simulink model "esercizio_3_massaMollaSmorzatore"  (R2024a)
settings: Solver=FixedStepAuto  StartTime=0.0  StopTime=15  RelTol=1e-3
PreLoadFcn:
  | clear %%pulisce il workspace
  | 
  | % --------------------
  | % system's parameters:
  | % --------------------
  | 
  | M = 5 % massa
  | M_nominal = M
  | K = 5 % costante elastica
  | K_nominal = K
  | S = 5 % costante smorzatore
  | S_nominal = S
  | 
  | N = 5 % numero giunti intere molla
  | L = 10 % lunghezza giunti
  | 
  | % --------------------
  | % desired eigenvalues
  | % --------------------
  | eig_H = 2*[-1 -2 ]
  | eig_G = 1*[-1 -2 ]
  | 
  | % --------------------
  | % matrix and initial conditions
  | % --------------------
  | A = [   0     1    ;
  |       -K/M  -S/M   ]
  | 
  | 
  | B = [  0  ;
  |       1/M ]
  | 
  | 
  | C = [0 1]
  | 
  | D = zeros(size(C,1),size(B,2))
  | 
  | 
  | dimx = size(A,1)  % quindi dimx = 2
  | dimu = size(B,2)  % quindi dimu = 1
  | dimy = size(C,1)  % quindi dimy = 1
  | 
  | x0 = [15; % posizione iniziale
  |       20] % velocità iniziale
  | % x0 = [0 0 0 0]'; %p.to di equilibrio
  | 
  | % --------------------
  | % certainty-equivalence state-feedback controller
  | % --------------------
  | G=place(A,B,eig_G) % costruisce matrice G dati gli autovalori desiderati
  | 
  | % --------------------
  | % Luenberger observer
  | % --------------------
  | 
  | %luenberger obs:
  | %  z_dot = Az + Bu + H(y-Cz) = (A-HC)z +[B H] [u y]
  | 
  | % initial conditions
  | z0 = [-.5; % posizione iniziale stimata
  |       -.31] % velocità iniziale stimata
  | 
  | %z0 = x0  %partenza con stima ok
  | 
  | H=place(A',C',eig_H)' % costruisce matrice H dati gli autovalori desiderati
  | 
  | A_lu = A-H*C
  | 
  | B_lu = [B H]
  | 
  | C_lu = eye(size(A))
  | 
  | D_lu = zeros(size(C_lu,1),size(B_lu,2))
InitFcn:
  | % --------------------
  | % matrix and initial conditions
  | % --------------------
  | A = [   0     1    ;
  |       -K_nominal/M_nominal  -S_nominal/M_nominal   ]
  | 
  | 
  | B = [  0  ;
  |       1/M_nominal ]
  | 
  | 
  | C = [ 0 1 ]
  | 
  | D = zeros(size(C,1),size(B,2))
  | 
  | % --------------------
  | % certainty-equivalence state-feedback controller
  | % --------------------
  | G=place(A,B,eig_G) % costruisce matrice G dati gli autovalori desiderati
  | 
  | % --------------------
  | % Luenberger observer
  | % --------------------
  | 
  | H=place(A',C',eig_H)' % costruisce matrice H dati gli autovalori desiderati
  | 
  | A_lu = A-H*C
  | 
  | B_lu = [B H]
  | 
  | C_lu = eye(size(A))
  | 
  | D_lu = zeros(size(C_lu,1),size(B_lu,2))
libraries: vrlib x14, sldrtlib x1
settings Model: Creator=39342  LastModifiedBy=39342

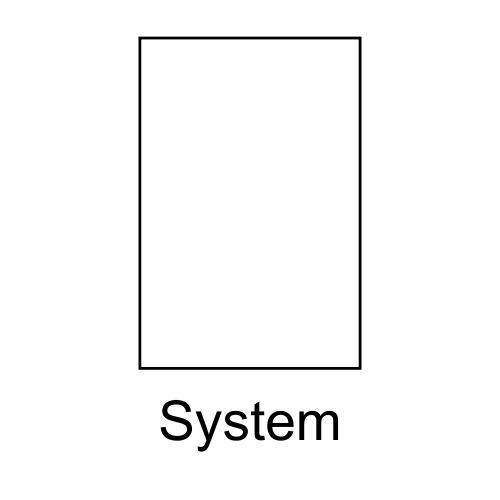
[thumbnail: Simulink's stored preview of the top-level diagram]
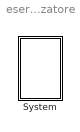
== system esercizio_3_massaMollaSmorzatore ==
  System : Subsystem

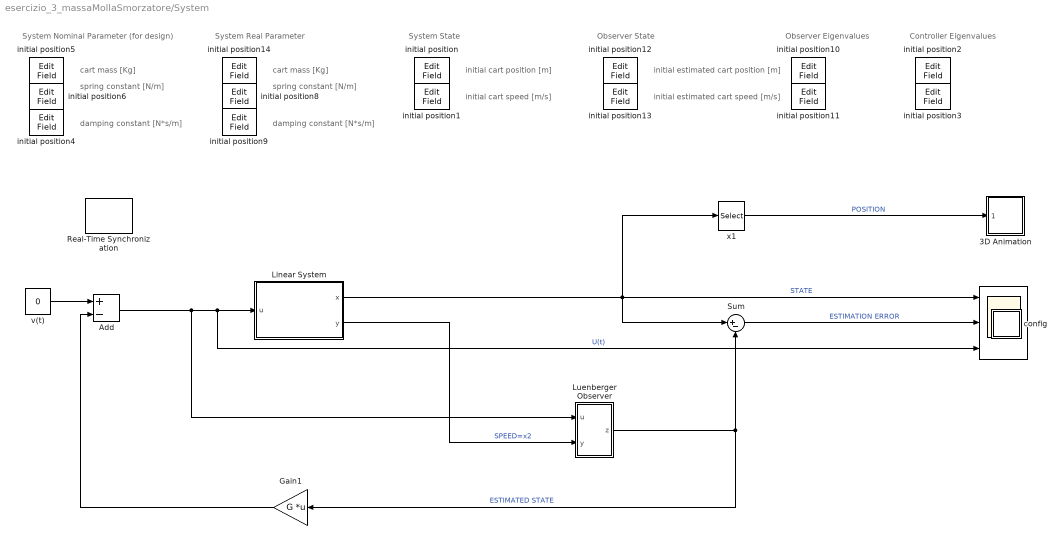
== system esercizio_3_massaMollaSmorzatore/System ==
  note: spring constant [N/m]
  note: initial estimated cart speed [m/s]
  note: System Real Parameter
  note: initial cart speed [m/s]
  note: cart mass [Kg]
  note: damping constant [N*s/m]
  note: initial cart position [m]
  note: Controller Eigenvalues
  note: cart mass [Kg]
  note: System State
  note: initial estimated cart position [m]
  note: damping constant [N*s/m]
  note: System Nominal Parameter (for design)
  note: Observer State
  note: Observer Eigenvalues
  note: spring constant [N/m]
  "     " : Scope  NumInputPorts=3
  3D Animation : Subsystem
  Add : Sum  Inputs=+-
  Gain1 : Gain  Gain=G  Multiplication=Matrix(K*u)
  Linear System : Subsystem
  Luenberger Observer : Subsystem
  Real-Time Synchronization : sldrtlib/Real-Time Synchronization  SampleTime=0.01  MaxMissedTicks=500  ShowMissedTicks=off  YieldWhenWaiting=off
  Sum : Sum  Inputs=|+-
  config : Subsystem
  initial position{,1..6,8..14} (14 alike) : EditField  LabelPosition=Hide  ShowInitialText=on  Alignment=Center
  v(t) : Constant  Value=0
  x1 : Selector  InputPortWidth=2  IndexOptions=Index vector (dialog)  Indices=[1]  OutputSizes=1
  wires:
  Sum/1 -> "     "/2  "ESTIMATION ERROR"
  x1/1 -> 3D Animation/1(position)  "POSITION"
  v(t)/1 -> Add/1
  Gain1/1 -> Add/2
  Luenberger Observer/1(z) -> Gain1/1, Sum/2  "ESTIMATED STATE"
  Linear System/1(x) -> Sum/1, "     "/1, x1/1  "STATE"
  Linear System/2(y) -> Luenberger Observer/2(y)  "SPEED=x2"
  Add/1 -> Linear System/1(u), "     "/3, Luenberger Observer/1(u)  "U(t)"

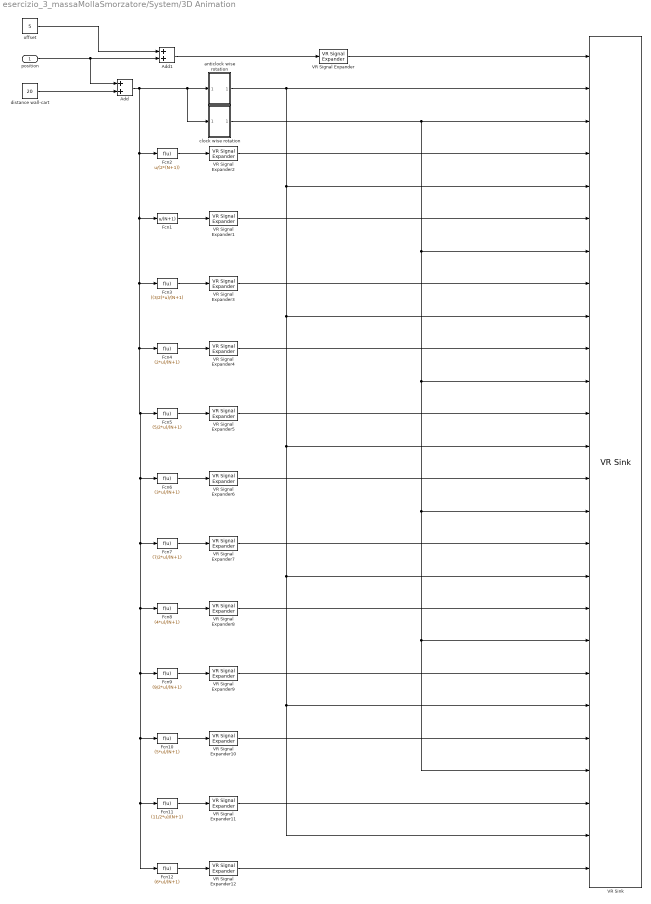
== system esercizio_3_massaMollaSmorzatore/System/3D Animation ==
  position : Inport
  Add : Sum
  Add1 : Sum
  Fcn1 : Fcn  Expr=u/(N+1)
  Fcn10 : Fcn  Expr=(5*u)/(N+1)
  Fcn11 : Fcn  Expr=(11/2*u)/(N+1)
  Fcn12 : Fcn  Expr=(6*u)/(N+1)
  Fcn2 : Fcn  Expr=u/(2*(N+1))
  Fcn3 : Fcn  Expr=((3/2)*u)/(N+1)
  Fcn4 : Fcn  Expr=(2*u)/(N+1)
  Fcn5 : Fcn  Expr=(5/2*u)/(N+1)
  Fcn6 : Fcn  Expr=(3*u)/(N+1)
  Fcn7 : Fcn  Expr=(7/2*u)/(N+1)
  Fcn8 : Fcn  Expr=(4*u)/(N+1)
  Fcn9 : Fcn  Expr=(9/2*u)/(N+1)
  VR Signal Expander{,1..12} (13 alike) : vrlib/VR Signal Expander  outwidth=3  outidx=[1]
  VR Sink : vrlib/VR Sink  InstantiateOnLoad=on  SampleTime=0.1  ViewEnable=on  RemoteChange=off  RemoteView=off  FieldsWritten=cart.translation.3.1.1.double#joint_1.rotation.4.1.1.double#joint_2.rotation.4.1.1.double#joint_2.translation.3.1.1.double#joint_3.rotation.4.1.1.double#joint_3.translation.3.1.1.double#joint_4.rotation.4.1.1.double#joint_4.translation.3.1.1.double#joint_5.rotation.4.1.1.double#joint_5.translation.3.1.1.double#joint_6.rotation.4.1.1.double#joint_6.translation.3.1.1.double#joint_7.rotation.4.1.1.double#joint_7.translation.3.1.1.double#joint_8.rotation.4.1.1.double#joint_8.translation.3.1.1.double#joint_9.rotation.4.1.1.double#joint_9.translation.3.1.1.double#joint_10.rotation.4.1.1.double#joint_10.translation.3.1.1.double#joint_11.rotation.4.1.1.double#joint_11.translation.3.1.1.double#joint_12.rotation.4.1.1.double#joint_12.translation.3.1.1.double#joint_13.rotation.4.1.1.double#joint_13.translation.3.1.1.double  WorldFileName=animazioneCarrello.x3d  AutoView=on  VideoDimensions=[]  AllowVariableSize=off
  anticlock wise rotation : Subsystem
  clock wise rotation : Subsystem
  distance wall-cart : Constant  Value=20
  offset : Constant  Value=5
  wires:
  position/1 -> Add1/2, Add/1
  distance wall-cart/1 -> Add/2
  Fcn2/1 -> VR Signal Expander2/1
  Fcn3/1 -> VR Signal Expander3/1
  Fcn4/1 -> VR Signal Expander4/1
  Fcn5/1 -> VR Signal Expander5/1
  Fcn6/1 -> VR Signal Expander6/1
  Fcn7/1 -> VR Signal Expander7/1
  Fcn8/1 -> VR Signal Expander8/1
  Fcn9/1 -> VR Signal Expander9/1
  VR Signal Expander/1 -> VR Sink/1
  anticlock wise rotation/1(Out1) -> VR Sink/25, VR Sink/21, VR Sink/17, VR Sink/13, VR Sink/9, VR Sink/5, VR Sink/2
  clock wise rotation/1(Out1) -> VR Sink/23, VR Sink/19, VR Sink/15, VR Sink/11, VR Sink/7, VR Sink/3
  VR Signal Expander2/1 -> VR Sink/4
  VR Signal Expander1/1 -> VR Sink/6
  VR Signal Expander3/1 -> VR Sink/8
  VR Signal Expander4/1 -> VR Sink/10
  VR Signal Expander5/1 -> VR Sink/12
  VR Signal Expander6/1 -> VR Sink/14
  VR Signal Expander7/1 -> VR Sink/16
  VR Signal Expander8/1 -> VR Sink/18
  VR Signal Expander9/1 -> VR Sink/20
  VR Signal Expander10/1 -> VR Sink/22
  Add/1 -> clock wise rotation/1(In1), anticlock wise rotation/1(In1), Fcn12/1, Fcn11/1, Fcn10/1, Fcn9/1, Fcn8/1, Fcn7/1, Fcn6/1, Fcn5/1, Fcn4/1, Fcn3/1, Fcn1/1, Fcn2/1
  Fcn10/1 -> VR Signal Expander10/1
  Fcn11/1 -> VR Signal Expander11/1
  VR Signal Expander11/1 -> VR Sink/24
  Fcn12/1 -> VR Signal Expander12/1
  VR Signal Expander12/1 -> VR Sink/26
  Fcn1/1 -> VR Signal Expander1/1
  Add1/1 -> VR Signal Expander/1
  offset/1 -> Add1/1

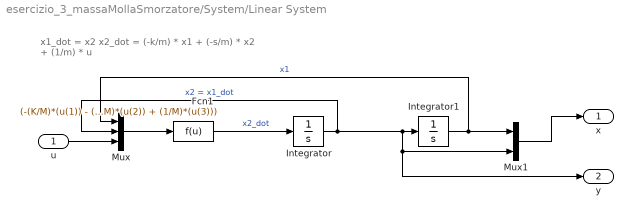
== system esercizio_3_massaMollaSmorzatore/System/Linear System ==
  note: x1_dot = x2
      | x2_dot = (-k/m) * x1 + (-s/m) * x2 + (1/m) * u
  u : Inport
  Fcn1 : Fcn  Expr=(-(K/M)*(u(1)) - (S/M)*(u(2)) + (1/M)*(u(3)))
  Integrator : Integrator  InitialCondition=x0(2)
  Integrator1 : Integrator  InitialCondition=x0(1)
  Mux : Mux  Inputs=3
  Mux1 : Mux  Inputs=2
  x : Outport
  y : Outport  Port=2
  wires:
  Fcn1/1 -> Integrator/1  "x2_dot"
  Integrator/1 -> Mux/2, y/1, Mux1/2, Integrator1/1  "x2 = x1_dot"
  Mux/1 -> Fcn1/1
  u/1 -> Mux/3
  Integrator1/1 -> Mux/1, Mux1/1  "x1"
  Mux1/1 -> x/1

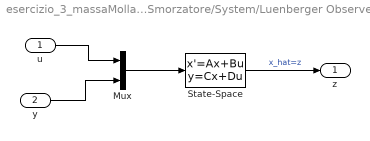
== system esercizio_3_massaMollaSmorzatore/System/Luenberger Observer ==
  u : Inport
  y : Inport  Port=2
  Mux : Mux  Inputs=2
  State-Space : StateSpace  A=A_lu  B=B_lu  C=C_lu  D=D_lu  InitialCondition=[z0(1); z0(2)]
  z : Outport
  wires:
  Mux/1 -> State-Space/1
  u/1 -> Mux/1
  State-Space/1 -> z/1  "x_hat=z"
  y/1 -> Mux/2

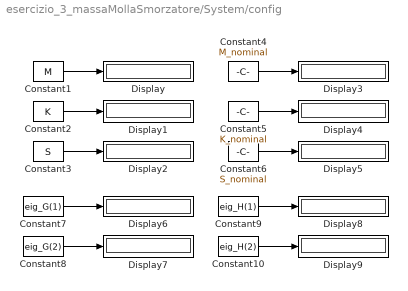
== system esercizio_3_massaMollaSmorzatore/System/config ==
  Constant1 : Constant  Value=M
  Constant10 : Constant  Value=eig_H(2)
  Constant2 : Constant  Value=K
  Constant3 : Constant  Value=S
  Constant4 : Constant  Value=M_nominal
  Constant5 : Constant  Value=K_nominal
  Constant6 : Constant  Value=S_nominal
  Constant7 : Constant  Value=eig_G(1)
  Constant8 : Constant  Value=eig_G(2)
  Constant9 : Constant  Value=eig_H(1)
  Display{,1..9} (10 alike) : Display
  wires:
  Constant7/1 -> Display6/1
  Constant1/1 -> Display/1
  Constant9/1 -> Display8/1
  Constant8/1 -> Display7/1
  Constant6/1 -> Display5/1
  Constant4/1 -> Display3/1
  Constant2/1 -> Display1/1
  Constant5/1 -> Display4/1
  Constant10/1 -> Display9/1
  Constant3/1 -> Display2/1

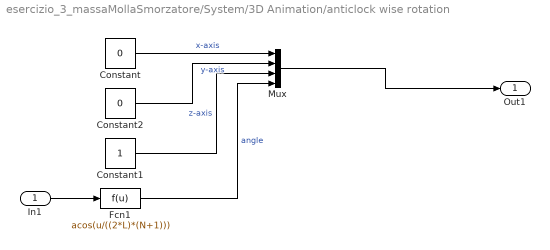
== system esercizio_3_massaMollaSmorzatore/System/3D Animation/anticlock wise rotation ==
  In1 : Inport
  Constant : Constant  Value=0
  Constant1 : Constant
  Constant2 : Constant  Value=0
  Fcn1 : Fcn  Expr=acos(u/((2*L)*(N+1)))
  Mux : Mux
  Out1 : Outport
  wires:
  Fcn1/1 -> Mux/4  "angle"
  Constant1/1 -> Mux/3  "z-axis"
  Constant2/1 -> Mux/2  "y-axis"
  Constant/1 -> Mux/1  "x-axis"
  In1/1 -> Fcn1/1
  Mux/1 -> Out1/1

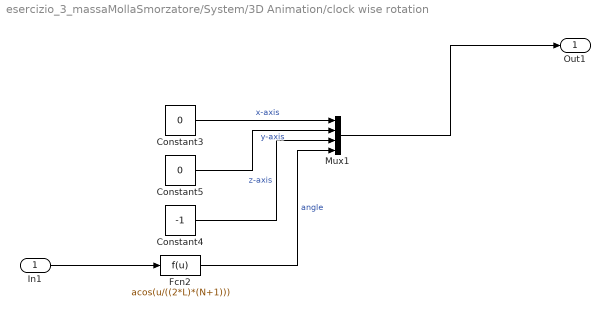
== system esercizio_3_massaMollaSmorzatore/System/3D Animation/clock wise rotation ==
  In1 : Inport
  Constant3 : Constant  Value=0
  Constant4 : Constant  Value=-1
  Constant5 : Constant  Value=0
  Fcn2 : Fcn  Expr=acos(u/((2*L)*(N+1)))
  Mux1 : Mux
  Out1 : Outport
  wires:
  Constant4/1 -> Mux1/3  "z-axis"
  Constant3/1 -> Mux1/1  "x-axis"
  Fcn2/1 -> Mux1/4  "angle"
  Constant5/1 -> Mux1/2  "y-axis"
  In1/1 -> Fcn2/1
  Mux1/1 -> Out1/1
